simulink model "Regelstrecke"  (R2025a)
settings: Solver=VariableStepAuto  StartTime=0.0  StopTime=10.0  RelTol=1e-3
model workspace (MATLAB code in the model file):
  | k = 1.380649e-23;
  | e = 1.602176634e-19;
  | T0 = 273.15;
  | 
  | UT = 26e-3;
  | IS = 1e-8;
  | R = 10e3;
  | L = 0.1;
  | C1 = 100e-9;
  | C2 = 1e-6;
  | 
  | U0_val = 12;
  | I0_val = 3e-3;
settings Model: Creator=richa  LastModifiedBy=richa

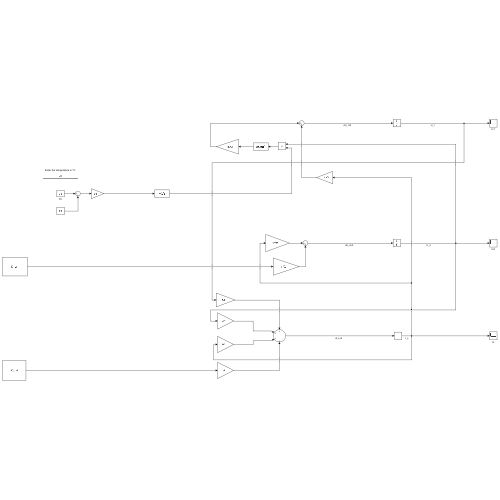
[thumbnail: Simulink's stored preview of the top-level diagram]
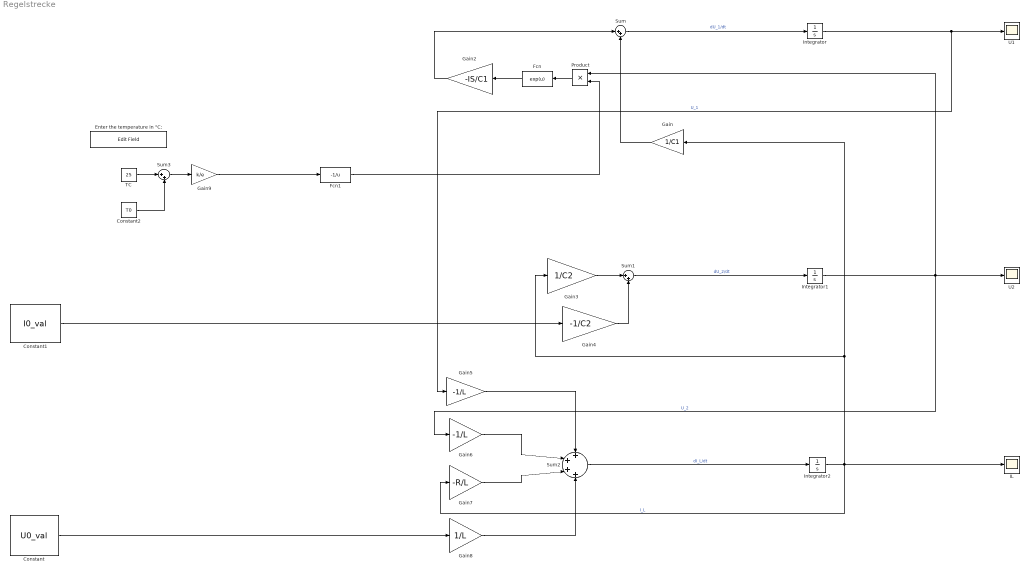
== system Regelstrecke ==
  Constant : Constant  Value=U0_val
  Constant1 : Constant  Value=I0_val
  Constant2 : Constant  Value=T0
  Enter the temperature in °C: : EditField  LabelPosition=Hide  ShowInitialText=on  Alignment=Center
  Fcn : Fcn  Expr=exp(u)
  Fcn1 : Fcn  Expr=-1/u
  Gain : Gain  Gain=1/C1
  Gain2 : Gain  Gain=-IS/C1
  Gain3 : Gain  Gain=1/C2
  Gain4 : Gain  Gain=-1/C2
  Gain5 : Gain  Gain=-1/L
  Gain6 : Gain  Gain=-1/L
  Gain7 : Gain  Gain=-R/L
  Gain8 : Gain  Gain=1/L
  Gain9 : Gain  Gain=k/e
  IL : Scope
      settings: DataLoggingVariableName=ScopeData2
  Integrator : Integrator
  Integrator1 : Integrator
  Integrator2 : Integrator
  Product : Product
  Sum : Sum  Inputs=|++
  Sum1 : Sum  Inputs=|++
  Sum2 : Sum  Inputs=++++
  Sum3 : Sum  Inputs=|++
  TC : Constant  Value=25
  U1 : Scope
  U2 : Scope
  wires:
  Integrator2/1 -> Gain7/1, IL/1, Gain3/1, Gain/1  "I_L"
  Gain/1 -> Sum/2
  Integrator1/1 -> U2/1, Product/1, Gain6/1  "U_2"
  Fcn/1 -> Gain2/1
  Gain2/1 -> Sum/1
  Sum/1 -> Integrator/1  "dU_1/dt"
  Gain3/1 -> Sum1/1
  Sum1/1 -> Integrator1/1  "dU_2/dt"
  Gain4/1 -> Sum1/2
  Constant1/1 -> Gain4/1
  Integrator/1 -> U1/1, Gain5/1  "U_1"
  Gain5/1 -> Sum2/1
  Gain6/1 -> Sum2/2
  Gain7/1 -> Sum2/3
  Gain8/1 -> Sum2/4
  Constant/1 -> Gain8/1
  Sum2/1 -> Integrator2/1  "dI_L/dt"
  Gain9/1 -> Fcn1/1
  Fcn1/1 -> Product/2
  Product/1 -> Fcn/1
  TC/1 -> Sum3/1
  Sum3/1 -> Gain9/1
  Constant2/1 -> Sum3/2
